simulink model "dcmtr_testharness"  (R2022b)
settings: Solver=ode15s  StartTime=0.0  StopTime=10  RelTol=1e-3
PostLoadFcn:
  | addpath GeneratedArtifacts/CodeGen
  | load('dcmtr_params');
undefined symbols (not defined in the file or in its folder): Ts
libraries: SignalEditorBlockLib x1
settings Model: Creator=smuckati  LastModifiedBy=smuckati
settings OptimizationCC: DefaultParameterBehavior=Inlined  UseDivisionForNetSlopeComputation=on  EnhancedBackFolding=on  PassReuseOutputArgsAs=Individual arguments  ZeroExternalMemoryAtStartup=off  ZeroInternalMemoryAtStartup=off  OptimizeBlockOrder=speed  DifferentSizesBufferReuse=on  OptimizationCustomize=off  EfficientTunableParamExpr=on
settings DebuggingCC: SignalRangeChecking=error  ParameterPrecisionLossMsg=none  ParameterTunabilityLossMsg=error  UnconnectedInputMsg=warning  UnconnectedOutputMsg=warning  UnconnectedLineMsg=warning
settings ModelReferenceCC: EnableRefExpFcnMdlSchedulingChecks=on
settings SFSimCC: MATLABDynamicMemAlloc=off
settings RTWCC: Description=Embedded Coder  SystemTargetFile=ert.tlc  GenCodeOnly=on  TemplateMakefile=ert_default_tmf  CodeExecutionProfiling=on  CodeProfilingSaveOptions=AllData  CodeProfilingInstrumentation=detailed  DLArmComputeVersion=19.05
settings CodeAppCC: ForceParamTrailComments=on  IgnoreCustomStorageClasses=off  OperatorAnnotations=on  SimulinkDataObjDesc=on  SFDataObjDesc=on  InsertBlockDesc=on
settings ERTTargetCC: TargetLangStandard=C99 (ISO)  GenerateSampleERTMain=on  InlinedParameterPlacement=NonHierarchical  ERTCustomFileTemplate=example_file_process.tlc

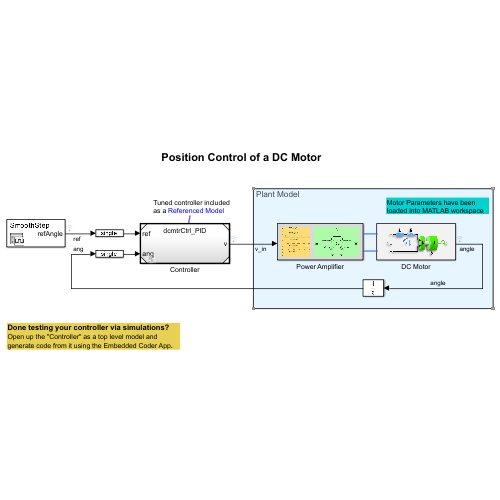
[thumbnail: Simulink's stored preview of the top-level diagram]
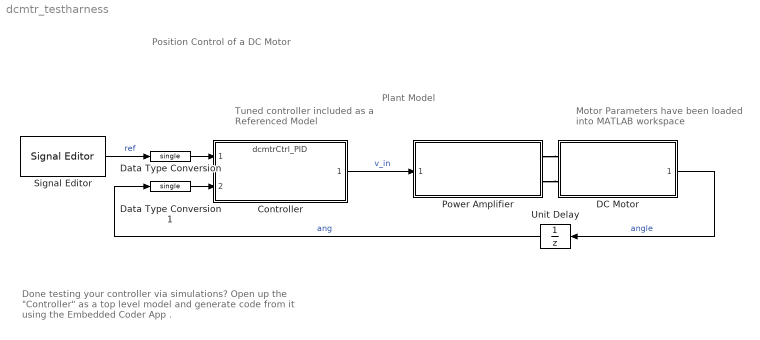
== system dcmtr_testharness ==
  note: Done testing your controller via simulations?
      | Open up the "Controller" as a top level model and generate code from it using the Embedded Coder App .
  note: Plant Model
  note: Motor Parameters have been loaded into MATLAB workspace
  note: Position Control of a DC Motor
  note: Tuned controller included as a Referenced Model
  Controller : ModelReference  ModelNameDialog=dcmtrCtrl_PID  SimulationMode=Normal  ModelReferenceVersion=3.0
  DC Motor : Subsystem  ReferencedSubsystem=dcmtr
  Data Type Conversion : DataTypeConversion  OutDataTypeStr=single  SaturateOnIntegerOverflow=off  RndMeth=Floor
  Data Type Conversion1 : DataTypeConversion  OutDataTypeStr=single  SaturateOnIntegerOverflow=off  RndMeth=Floor
  Power Amplifier : Subsystem  ReferencedSubsystem=powerAmp
  Signal Editor : SignalEditorBlockLib/Signal Editor  FileName=dcmtrCtrl_testRefAngles.mat  ActiveScenario=SmoothStep  ActiveSignal=refAngle  IsBus=off  OutputBusObjectStr=Bus: BusObject  SampleTime=0  ZeroCross=off  OutputAfterFinalValue=Setting to zero  Unit=inherit  PreserveSignalName=on
  Unit Delay : UnitDelay  SampleTime=Ts  HasFrameUpgradeWarning=on
  wires:
  DC Motor/1 -> Unit Delay/1  "angle"
  Signal Editor/1 -> Data Type Conversion/1  "ref"
  Unit Delay/1 -> Data Type Conversion1/1  "ang"
  Controller/1 -> Power Amplifier/1  "v_in"
  Data Type Conversion/1 -> Controller/1
  Data Type Conversion1/1 -> Controller/2
  connections:
  Power Amplifier/RConn1 -- DC Motor/LConn1
  Power Amplifier/RConn2 -- DC Motor/LConn2
